simulink library "SEL751_SignalScaling_lib"  (Simulink 8.1)
settings: Solver=ode45  StartTime=0.0  StopTime=10.0  RelTol=1e-3
settings Model: Creator=RE25624  LastModifiedBy=RE25624

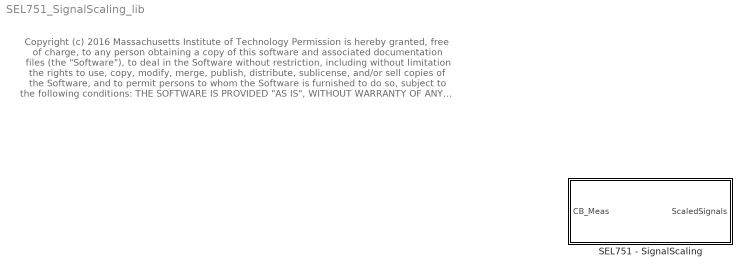
== system SEL751_SignalScaling_lib ==
  note: Copyright (c) 2016 Massachusetts Institute of Technology
      | Permission is hereby granted, free of charge, to any person obtaining a copy of this software and associated documentation files (the "Software"), to deal
      | in the Software without restriction, including without limitation the rights to use, copy, modify, merge, publish, distribute, sublicense, and/or sell copies of the
      | Software, and to permit persons to whom the Software is furnished to do so, subject to the following conditions:
      |
      | THE SOFTWARE IS PROVIDED "AS IS", WITHOUT WARRANTY OF ANY KIND, EXPRESS OR IMPLIED, INCLUDING BUT NOT LIMITED TO THE
      | WARRANTIES OF MERCHANTABILITY, FITNESS FOR A PARTICULAR PURPOSE AND NONINFRINGEMENT. IN NO EVENT SHALL THE AUTHORS
      | OR COPYRIGHT HOLDERS BE LIABLE FOR ANY CLAIM, DAMAGES OR OTHER LIABILITY, WHETHER IN AN ACTION OF CONTRACT, TORT OR
      | OTHERWISE, ARISING FROM, OUT OF OR IN CONNECTION WITH THE SOFTWARE OR THE USE OR OTHER DEALINGS IN THE SOFTWARE
  SEL751 - SignalScaling : Subsystem  mask(SEL751 - SignalScaling){ct_ratio=5/1250, pt_ratio=1/1800}
      mask prompts: ct_ratio "CT Ratio"; pt_ratio "PT Ratio"

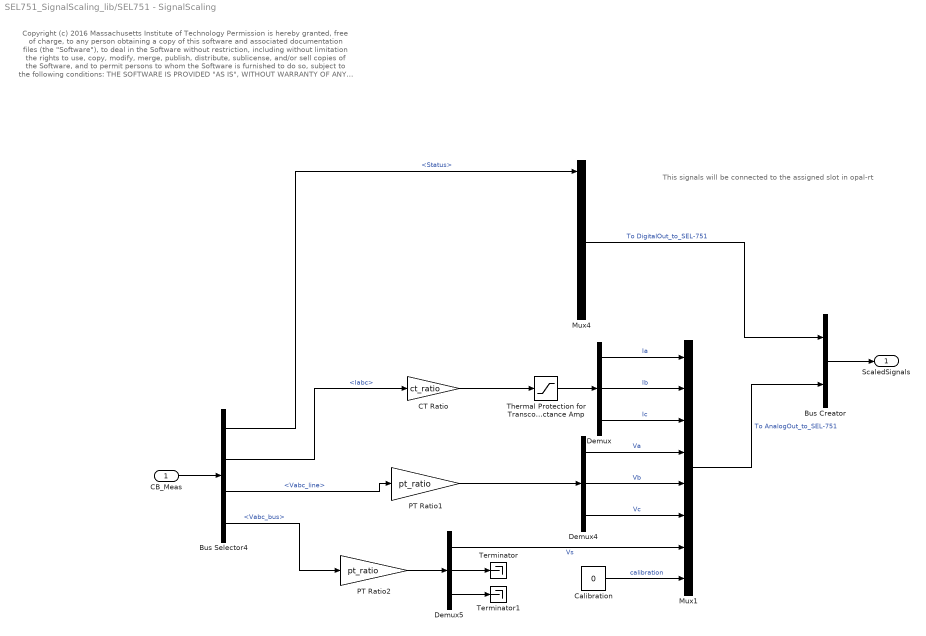
== system SEL751_SignalScaling_lib/SEL751 - SignalScaling ==
  note: Copyright (c) 2016 Massachusetts Institute of Technology
      | Permission is hereby granted, free of charge, to any person obtaining a copy of this software and associated documentation files (the "Software"), to deal
      | in the Software without restriction, including without limitation the rights to use, copy, modify, merge, publish, distribute, sublicense, and/or sell copies of the
      | Software, and to permit persons to whom the Software is furnished to do so, subject to the following conditions:
      |
      | THE SOFTWARE IS PROVIDED "AS IS", WITHOUT WARRANTY OF ANY KIND, EXPRESS OR IMPLIED, INCLUDING BUT NOT LIMITED TO THE
      | WARRANTIES OF MERCHANTABILITY, FITNESS FOR A PARTICULAR PURPOSE AND NONINFRINGEMENT. IN NO EVENT SHALL THE AUTHORS
      | OR COPYRIGHT HOLDERS BE LIABLE FOR ANY CLAIM, DAMAGES OR OTHER LIABILITY, WHETHER IN AN ACTION OF CONTRACT, TORT OR
      | OTHERWISE, ARISING FROM, OUT OF OR IN CONNECTION WITH THE SOFTWARE OR THE USE OR OTHER DEALINGS IN THE SOFTWARE
  note: This signals will be connected to the assigned slot in opal-rt
  CB_Meas : Inport
  Bus Creator : BusCreator  Inputs=2
  Bus Selector4 : BusSelector  OutputSignals=Status,Iabc,Vabc_line,Vabc_bus
  CT Ratio : Gain  Gain=ct_ratio
  Calibration : Constant  Value=0
  Demux : Demux  Outputs=3
  Demux4 : Demux  Outputs=3
  Demux5 : Demux  Outputs=3
  Mux1 : Mux  Inputs=8
  Mux4 : Mux  Inputs=8
  PT Ratio1 : Gain  Gain=pt_ratio
  PT Ratio2 : Gain  Gain=pt_ratio
  Terminator : Terminator
  Terminator1 : Terminator
  Thermal Protection for Transconductance Amp : Saturate  UpperLimit=5  LowerLimit=-5
  ScaledSignals : Outport
  wires:
  Bus Creator/1 -> ScaledSignals/1
  Demux5/3 -> Terminator1/1
  Demux5/2 -> Terminator/1
  Thermal Protection for Transconductance Amp/1 -> Demux/1
  PT Ratio2/1 -> Demux5/1
  PT Ratio1/1 -> Demux4/1
  CT Ratio/1 -> Thermal Protection for Transconductance Amp/1
  CB_Meas/1 -> Bus Selector4/1
  Demux/2 -> Mux1/2  "Ib"
  Demux/3 -> Mux1/3  "Ic"
  Demux/1 -> Mux1/1  "Ia"
  Mux1/1 -> Bus Creator/2  "To AnalogOut_to_SEL-751"
  Mux4/1 -> Bus Creator/1  "To DigitalOut_to_SEL-751"
  Bus Selector4/1 -> Mux4/1  "<Status>"
  Calibration/1 -> Mux1/8  "calibration"
  Bus Selector4/3 -> PT Ratio1/1  "<Vabc_line>"
  Demux5/1 -> Mux1/7  "Vs"
  Bus Selector4/4 -> PT Ratio2/1  "<Vabc_bus>"
  Demux4/3 -> Mux1/6  "Vc"
  Demux4/2 -> Mux1/5  "Vb"
  Demux4/1 -> Mux1/4  "Va"
  Bus Selector4/2 -> CT Ratio/1  "<Iabc>"
